simulink model "Microgrid"  (R2022b)
settings: Solver=ode45  StartTime=0.0  StopTime=0.5  RelTol=1e-3  EnableMultiTasking=on
model workspace (MAT data in the model file):
  AFPV = 1
  AFW = 1
  DG = 1
  pvc = 1
  wf1 = 1
undefined symbols (not defined in the file): BMSS1, D1, Delta, Ion, Lithium, R
libraries: spsDiodeLib x10, spsVoltageMeasurementLib x8, spsThreePhaseVIMeasurementLib x7, spsSeriesRLCBranchLib x7, fuzblock x6, spsMosfetLib x3, powerlib_extras x3, spsBreakerLib x2, spsThreePhaseParallelRLCLoadLib x2, spsThreePhaseBreakerLib x2, spsPWMGenerator2LevelLib x2, spsBatteryLib x1
(part 1 of 2)
settings Model: Creator=Indhu  LastModifiedBy=zs
settings SolverCC: AlgebraicLoopSolver=TrustRegion
settings DataIOCC: LimitDataPoints=on  SaveFormat=Array  ReturnWorkspaceOutputs=off
settings OptimizationCC: LifeSpan=inf
settings DebuggingCC: SolverPrmCheckMsg=warning  UnconnectedInputMsg=warning  UnconnectedOutputMsg=warning  UnconnectedLineMsg=warning  SFUnexpectedBacktrackingDiag=warning  SFNoUnconditionalDefaultTransitionDiag=warning  SFExecutionAtInitializationDiag=none  SFMachineParentedDataDiag=warning  ArithmeticOperatorsInVariantConditions=warning
settings HardwareCC: ProdBitPerPointer=32  ProdBitPerSizeT=32  ProdBitPerPtrDiffT=32  ProdLargestAtomicFloat=None  ProdIntDivRoundTo=Undefined  ProdEndianess=Unspecified  ProdWordSize=32  ProdHWDeviceType=32-bit Generic
settings ModelReferenceCC: EnableRefExpFcnMdlSchedulingChecks=on  PropagateSignalLabelsOutOfModel=off
settings SFSimCC: SimUseLocalCustomCode=off  CustomCodeUndefinedFunction=UseInterfaceOnly
settings RTWCC: RTWUseLocalCustomCode=off
settings CodeAppCC: StateflowObjectComments=on
settings GRTTargetCC: TargetLangStandard=C89/C90 (ANSI)
settings ConfigComp: CovMetricSettings=dw  CovSaveCumulativeToWorkspaceVar=on  CovSaveSingleToWorkspaceVar=on  CovExternalEMLEnable=off  CovSFcnEnable=off
settings SimscapeCC: SimscapeNormalizeSystem=off

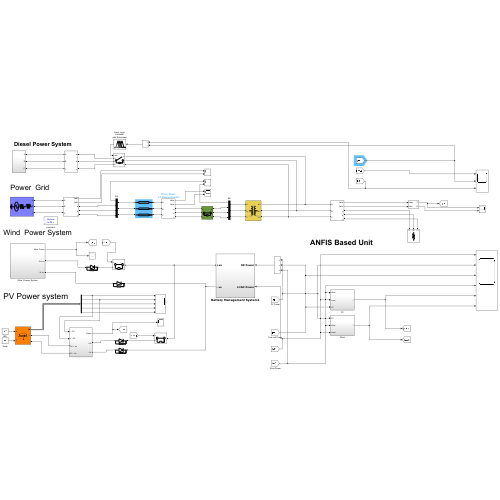
[thumbnail: Simulink's stored preview of the top-level diagram]
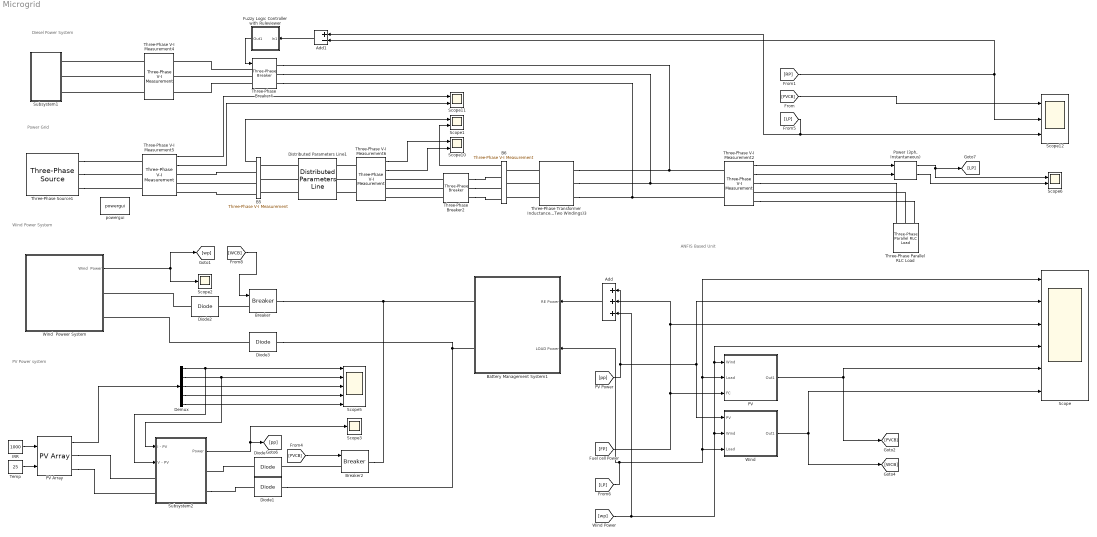
== system Microgrid ==
  note: ANFIS Based Unit
  note: Power Grid
  note: Wind Power System
  note: PV Power system
  note: Diesel Power System
  Add : Sum  Inputs=+++
  Add1 : Sum  Inputs=+-
  B5 : spsThreePhaseVIMeasurementLib/Three-Phase V-I Measurement  VoltageMeasurement=phase-to-ground  SetLabelV=off  LabelV=Vabc_B12  Vpu=off  VpuLL=off  CurrentMeasurement=no  SetLabelI=off  LabelI=A1  Ipu=off  Pbase=100e6  Vbase=25e3  OutputType=Magnitude  PhasorSimulation=off  PSBequivalent=0
  B6 : spsThreePhaseVIMeasurementLib/Three-Phase V-I Measurement  VoltageMeasurement=phase-to-phase  SetLabelV=off  LabelV=Vabc_B12  Vpu=off  VpuLL=off  CurrentMeasurement=no  SetLabelI=off  LabelI=A1  Ipu=off  Pbase=100e6  Vbase=440  OutputType=Magnitude  PhasorSimulation=off  PSBequivalent=0
  Battery Management System1 : Subsystem
  Breaker : spsBreakerLib/Breaker  InitialState=1  SwitchingTimes="[1/60  5/60]"  External=on  BreakerResistance=0.01  SnubberResistance=1e6  SnubberCapacitance=inf  Measurements=None  MoreParameters=on  NoBreakLoop=off
  Breaker2 : spsBreakerLib/Breaker  InitialState=1  SwitchingTimes="[1/60  5/60]"  External=on  BreakerResistance=0.01  SnubberResistance=1e6  SnubberCapacitance=inf  Measurements=None  MoreParameters=on  NoBreakLoop=off
  Demux : Demux  Outputs=5
  Diode{,1..3} (4 alike) : spsDiodeLib/Diode  Ron=0.001  Lon=0  Vf=0.8  IC=0  UseSnubber=off  Rs=500  Cs=250e-9  Measurements=off
  Distributed Parameters Line1 : spsDistributedParametersLineLib/Distributed Parameters Line  Phases=3  Length=100  Frequency=50  Resistance=[0.01273 0.3864]  Inductance="[0.9337e-3  4.1264e-3]"  Capacitance=[12.74e-9 7.751e-9]  x1=[-0.000566 2.77076590585873e-09 21709.9833530794 -60790.4116423668;-0.000565 2.76912057824268e-09 21729.080152483 -60783.5882501713;-0.000564 2.76747497732538e-09 21748.1748073123 -60776.7588588762;-0.000563 2.76582910326925e-09 21767.2673156828 -60769.9234691554;-0.000562 2.76418295623673e-09 21786.3576757102 -60763.0820816836;-0.000561 2.76253653639029e-09 21805.4458855103 -60756.234697136;-0.00056 2.76088984389243e-09 21824.5319431991 -60749.3813161885;-0.000559 2.75924287890566e-09 21843.615846893 -60742.5219395174;-0.000558 2.75759564159254e-09 21862.6975947085 -60735.6565677998;-0.000557 2.75594813211564e-09 21881.7771847622 -60728.7852017131;-0.000556 2.75430035063756e-09 21900.8546151711 -60721.9078419357;-0.000555 2.75265229732094e-09 21919.9298840522 -60715.0244891462;-0.000554 2.75100397232843e-09 21939.0029895231 -60708.1351440241;-0.000553 2.74935537582271e-09 21958.0739297011 -60701.2398072492;-0.000552 2.74770650796649e-09 21977.1427027041 -60694.3384795021;-0.000551 2.74605736892252e-09 21996.2093066501 -60687.431161464;-0.00055 2.74440795885354e-09 22015.2737396573 -60680.5178538165;-0.000549 2.74275827792236e-09 22034.3359998441 -60673.598557242;-0.000548 2.74110832629179e-09 22053.3960853291 -60666.6732724235;-0.000547 2.73945810412468e-09 22072.4539942312 -60659.7420000443;-0.000546 2.73780761158389e-09 22091.5097246694 -60652.8047407886;-0.000545 2.73615684883232e-09 22110.5632747629 -60645.8614953411;-0.000544 2.7345058160329e-09 22129.6146426314 -60638.912264387;-0.000543 2.73285451334857e-09 22148.6638263945 -60631.9570486122;-0.000542 2.73120294094231e-09 22167.7108241721 -60624.9958487031;-0.000541 2.72955109897714e-09 22186.7556340844 -60618.0286653468;-0.00054 2.72789898761607e-09 22205.7982542516 -60611.055499231;-0.000539 2.72624660702216e-09 22224.8386827945 -60604.0763510438;-0.000538 2.7245939573585e-09 22243.8769178337 -60597.0912214741;-0.000537 2.72294103878819e-09 22262.9129574902 -60590.1001112112;-0.000536 2.72128785147438e-09 22281.9467998854 -60583.1030209452;-0.000535 2.71963439558023e-09 22300.9784431405 -60576.0999513666;-0.000534 2.71798067126893e-09 22320.0078853774 -60569.0909031667;-0.000533 2.71632667870368e-09 22339.0351247177 -60562.0758770372;-0.000532 2.71467241804774e-09 22358.0601592837 -60555.0548736704;-0.000531 2.71301788946438e-09 22377.0829871976 -60548.0278937593;-0.00053 2.71136309311688e-09 22396.103606582 -60540.9949379974;-0.000529 2.70970802916857e-09 22415.1220155596 -60533.9560070788;-0.000528 2.70805269778281e-09 22434.1382122533 -60526.9111016984;-0.000527 2.70639709912295e-09 22453.1521947863 -60519.8602225512;-0.000526 2.70474123335242e-09 22472.1639612821 -60512.8033703334;-0.000525 2.70308510063462e-09 22491.1735098642 -60505.7405457413;-0.000524 2.70142870113302e-09 22510.1808386564 -60498.671749472;-0.000523 2.6997720350111e-09 22529.1859457829 -60491.5969822232;-0.000522 2.69811510243236e-09 22548.1888293679 -60484.5162446931;-0.000521 2.69645790356033e-09 22567.1894875358 -60477.4295375806;-0.00052 2.69480043855858e-09 22586.1879184115 -60470.3368615851;-0.000519 2.69314270759069e-09 22605.1841201197 -60463.2382174066;-0.000518 2.69148471082027e-09 22624.1780907858 -60456.1336057458;-0.000517 2.68982644841096e-09 22643.1698285349 -60449.0230273037;-0.000516 2.68816792052642e-09 22662.1593314929 -60441.9064827823;-0.000515 2.68650912733035e-09 22681.1465977853 -60434.7839728839;-0.000514 2.68485006898645e-09 22700.1316255383 -60427.6554983114;-0.000513 2.68319074565847e-09 22719.1144128782 -60420.5210597684;-0.000512 2.68153115751019e-09 22738.0949579314 -60413.3806579591;-0.000511 2.67987130470539e-09 22757.0732588245 -60406.2342935881;-0.00051 2.67821118740789e-09 22776.0493136846 -60399.0819673609;-0.000509 2.67655080578155e-09 22795.0231206387 -60391.9236799832;-0.000508 2.67489015999024e-09 22813.9946778142 -60384.7594321616;-0.000507 2.67322925019785e-09 22832.9639833388 -60377.5892246032;-0.000506 2.67156807656831e-09 22851.9310353401 ...(+33013 chars)]  x2=[-0.000566 1.4309886308804e-08 21803.469224195 -61159.1015753649;-0.000565 1.43032919359107e-08 21822.6818463418 -61152.2487955231;-0.000564 1.42966961513391e-08 21841.8923146763 -61145.3899801964;-0.000563 1.42900989557401e-08 21861.1006273024 -61138.5251300616;-0.000562 1.4283500349765e-08 21880.3067823244 -61131.6542457963;-0.000561 1.42769003340648e-08 21899.5107778466 -61124.7773280786;-0.00056 1.42702989092911e-08 21918.7126119739 -61117.8943775873;-0.000559 1.42636960760953e-08 21937.9122828109 -61111.0053950016;-0.000558 1.42570918351292e-08 21957.1097884627 -61104.1103810014;-0.000557 1.42504861870445e-08 21976.3051270348 -61097.2093362674;-0.000556 1.42438791324932e-08 21995.4982966324 -61090.3022614805;-0.000555 1.42372706721274e-08 22014.6892953614 -61083.3891573226;-0.000554 1.42306608065993e-08 22033.8781213277 -61076.4700244758;-0.000553 1.42240495365613e-08 22053.0647726374 -61069.5448636231;-0.000552 1.42174368626659e-08 22072.2492473968 -61062.6136754479;-0.000551 1.42108227855658e-08 22091.4315437126 -61055.6764606344;-0.00055 1.42042073059136e-08 22110.6116596915 -61048.7332198672;-0.000549 1.41975904243625e-08 22129.7895934406 -61041.7839538316;-0.000548 1.41909721415653e-08 22148.9653430669 -61034.8286632135;-0.000547 1.41843524581753e-08 22168.138906678 -61027.8673486993;-0.000546 1.41777313748458e-08 22187.3102823816 -61020.900010976;-0.000545 1.41711088922304e-08 22206.4794682854 -61013.9266507313;-0.000544 1.41644850109825e-08 22225.6464624975 -61006.9472686536;-0.000543 1.41578597317561e-08 22244.8112631263 -60999.9618654315;-0.000542 1.41512330552049e-08 22263.9738682802 -60992.9704417545;-0.000541 1.4144604981983e-08 22283.134276068 -60985.9729983127;-0.00054 1.41379755127446e-08 22302.2924845986 -60978.9695357967;-0.000539 1.41313446481439e-08 22321.4484919811 -60971.9600548976;-0.000538 1.41247123888354e-08 22340.6022963251 -60964.9445563074;-0.000537 1.41180787354737e-08 22359.75389574 -60957.9230407183;-0.000536 1.41114436887135e-08 22378.9032883356 -60950.8955088235;-0.000535 1.41048072492097e-08 22398.0504722221 -60943.8619613164;-0.000534 1.40981694176171e-08 22417.1954455096 -60936.8223988913;-0.000533 1.40915301945911e-08 22436.3382063086 -60929.7768222429;-0.000532 1.40848895807867e-08 22455.4787527297 -60922.7252320667;-0.000531 1.40782475768595e-08 22474.617082884 -60915.6676290585;-0.00053 1.4071604183465e-08 22493.7531948826 -60908.604013915;-0.000529 1.40649594012588e-08 22512.8870868366 -60901.5343873333;-0.000528 1.40583132308967e-08 22532.0187568578 -60894.4587500111;-0.000527 1.40516656730348e-08 22551.1482030579 -60887.3771026467;-0.000526 1.40450167283291e-08 22570.2754235489 -60880.2894459392;-0.000525 1.40383663974358e-08 22589.4004164431 -60873.1957805879;-0.000524 1.40317146810112e-08 22608.5231798528 -60866.0961072932;-0.000523 1.4025061579712e-08 22627.6437118907 -60858.9904267555;-0.000522 1.40184070941947e-08 22646.7620106697 -60851.8787396764;-0.000521 1.4011751225116e-08 22665.8780743029 -60844.7610467575;-0.00052 1.4005093973133e-08 22684.9919009036 -60837.6373487015;-0.000519 1.39984353389026e-08 22704.1034885854 -60830.5076462114;-0.000518 1.3991775323082e-08 22723.212835462 -60823.3719399909;-0.000517 1.39851139263285e-08 22742.3199396474 -60816.2302307443;-0.000516 1.39784511492997e-08 22761.4247992558 -60809.0825191764;-0.000515 1.3971786992653e-08 22780.5274124017 -60801.9288059926;-0.000514 1.39651214570463e-08 22799.6277771996 -60794.7690918991;-0.000513 1.39584545431373e-08 22818.7258917645 -60787.6033776024;-0.000512 1.3951786251584e-08 22837.8217542114 -60780.4316638097;-0.000511 1.39451165830447e-08 22856.9153626557 -60773.253951229;-0.00051 1.39384455381776e-08 22876.0067152129 -60766.0702405685;-0.000509 1.3931773117641e-08 22895.0958099987 -60758.8805325374;-0.000508 1.39250993220935e-08 22914.1826451292 -60751.6848278452;-0.000507 1.39184241521939e-08 22933.2672187205 -60744.483127202;-0.000506 1.39117476086008e-08 22952.3495288891 -60737.2754313188 ...(+32992 chars)]  x3=[-0.000566 1.37069561345331e-10 55.3596099410286 -231.821785243805;-0.000565 1.37082432995365e-10 55.4324361696897 -231.804382069755;-0.000564 1.37095291115906e-10 55.5052569273886 -231.786956017529;-0.000563 1.37108135705683e-10 55.5780722069384 -231.769507088848;-0.000562 1.3712096676343e-10 55.6508820011523 -231.752035285434;-0.000561 1.37133784287881e-10 55.7236863028444 -231.734540609011;-0.00056 1.37146588277769e-10 55.7964851048291 -231.717023061306;-0.000559 1.37159378731832e-10 55.8692783999215 -231.699482644048;-0.000558 1.37172155648806e-10 55.9420661809372 -231.681919358967;-0.000557 1.37184919027432e-10 56.0148484406923 -231.664333207798;-0.000556 1.37197668866449e-10 56.0876251720036 -231.646724192275;-0.000555 1.37210405164599e-10 56.1603963676881 -231.629092314138;-0.000554 1.37223127920625e-10 56.2331620205637 -231.611437575125;-0.000553 1.37235837133271e-10 56.3059221234488 -231.59375997698;-0.000552 1.37248532801283e-10 56.3786766691621 -231.576059521448;-0.000551 1.37261214923408e-10 56.4514256505231 -231.558336210274;-0.00055 1.37273883498394e-10 56.5241690603518 -231.54059004521;-0.000549 1.37286538524991e-10 56.5969068914686 -231.522821028005;-0.000548 1.3729918000195e-10 56.6696391366947 -231.505029160413;-0.000547 1.37311807928023e-10 56.7423657888516 -231.487214444191;-0.000546 1.37324422301964e-10 56.8150868407616 -231.469376881098;-0.000545 1.37337023122528e-10 56.8878022852472 -231.451516472892;-0.000544 1.37349610388471e-10 56.9605121151319 -231.433633221338;-0.000543 1.37362184098551e-10 57.0332163232394 -231.4157271282;-0.000542 1.37374744251527e-10 57.1059149023942 -231.397798195245;-0.000541 1.37387290846159e-10 57.1786078454211 -231.379846424243;-0.00054 1.37399823881209e-10 57.2512951451456 -231.361871816966;-0.000539 1.37412343355441e-10 57.3239767943938 -231.343874375187;-0.000538 1.37424849267617e-10 57.3966527859924 -231.325854100684;-0.000537 1.37437341616505e-10 57.4693231127684 -231.307810995234;-0.000536 1.37449820400871e-10 57.5419877675496 -231.289745060618;-0.000535 1.37462285619484e-10 57.6146467431644 -231.27165629862;-0.000534 1.37474737271113e-10 57.6873000324414 -231.253544711024;-0.000533 1.37487175354529e-10 57.7599476282102 -231.235410299618;-0.000532 1.37499599868505e-10 57.8325895233007 -231.217253066193;-0.000531 1.37512010811815e-10 57.9052257105435 -231.199073012539;-0.00053 1.37524408183233e-10 57.9778561827696 -231.180870140452;-0.000529 1.37536791981537e-10 58.0504809328107 -231.162644451727;-0.000528 1.37549162205503e-10 58.123099953499 -231.144395948165;-0.000527 1.37561518853911e-10 58.1957132376674 -231.126124631564;-0.000526 1.37573861925542e-10 58.2683207781491 -231.10783050373;-0.000525 1.37586191419176e-10 58.3409225677781 -231.089513566468;-0.000524 1.37598507333598e-10 58.4135185993889 -231.071173821585;-0.000523 1.37610809667592e-10 58.4861088658166 -231.052811270891;-0.000522 1.37623098419944e-10 58.5586933598967 -231.034425916199;-0.000521 1.3763537358944e-10 58.6312720744655 -231.016017759323;-0.00052 1.37647635174869e-10 58.7038450023597 -230.997586802081;-0.000519 1.37659883175022e-10 58.7764121364167 -230.979133046291;-0.000518 1.37672117588688e-10 58.8489734694744 -230.960656493774;-0.000517 1.37684338414662e-10 58.9215289943713 -230.942157146354;-0.000516 1.37696545651736e-10 58.9940787039464 -230.923635005857;-0.000515 1.37708739298705e-10 59.0666225910393 -230.905090074112;-0.000514 1.37720919354367e-10 59.1391606484903 -230.886522352947;-0.000513 1.3773308581752e-10 59.2116928691402 -230.867931844196;-0.000512 1.37745238686961e-10 59.2842192458303 -230.849318549694;-0.000511 1.37757377961493e-10 59.3567397714025 -230.830682471277;-0.00051 1.37769503639917e-10 59.4292544386993 -230.812023610786;-0.000509 1.37781615721035e-10 59.5017632405639 -230.793341970061;-0.000508 1.37793714203654e-10 59.5742661698399 -230.774637550946;-0.000507 1.37805799086578e-10 59.6467632193716 -230.755910355288;-0.000506 1.37817870368614e-10 59.7192543820037 ...(+33006 chars)]  x4=[-0.000566 -1.1176625836894e-10 80.4359037202969 -225.752108293466;-0.000565 -1.11789344885578e-10 80.5068218662724 -225.72682746904;-0.000564 -1.11812420369049e-10 80.5777320665431 -225.70152436627;-0.000563 -1.11835484817077e-10 80.6486343141105 -225.676198987652;-0.000562 -1.11858538227385e-10 80.7195286019768 -225.650851335687;-0.000561 -1.11881580597698e-10 80.790414923145 -225.625481412875;-0.00056 -1.11904611925742e-10 80.861293270619 -225.600089221721;-0.000559 -1.11927632209243e-10 80.9321636374032 -225.574674764731;-0.000558 -1.1195064144593e-10 81.0030260165031 -225.549238044413;-0.000557 -1.11973639633531e-10 81.0738804009249 -225.523779063278;-0.000556 -1.11996626769778e-10 81.1447267836754 -225.498297823838;-0.000555 -1.120196028524e-10 81.2155651577625 -225.472794328608;-0.000554 -1.12042567879131e-10 81.2863955161947 -225.447268580106;-0.000553 -1.12065521847704e-10 81.3572178519813 -225.42172058085;-0.000552 -1.12088464755853e-10 81.4280321581323 -225.396150333363;-0.000551 -1.12111396601314e-10 81.4988384276588 -225.370557840167;-0.00055 -1.12134317381824e-10 81.5696366535725 -225.344943103789;-0.000549 -1.1215722709512e-10 81.6404268288857 -225.319306126757;-0.000548 -1.12180125738942e-10 81.7112089466118 -225.293646911601;-0.000547 -1.1220301331103e-10 81.781982999765 -225.267965460853;-0.000546 -1.12225889809124e-10 81.85274898136 -225.242261777048;-0.000545 -1.12248755230966e-10 81.9235068844125 -225.216535862724;-0.000544 -1.12271609574301e-10 81.9942567019392 -225.190787720418;-0.000543 -1.12294452836872e-10 82.064998426957 -225.165017352673;-0.000542 -1.12317285016425e-10 82.1357320524843 -225.139224762031;-0.000541 -1.12340106110707e-10 82.2064575715398 -225.113409951039;-0.00054 -1.12362916117464e-10 82.2771749771432 -225.087572922244;-0.000539 -1.12385715034446e-10 82.347884262315 -225.061713678196;-0.000538 -1.12408502859403e-10 82.4185854200764 -225.035832221448;-0.000537 -1.12431279590085e-10 82.4892784434496 -225.009928554553;-0.000536 -1.12454045224245e-10 82.5599633254574 -224.984002680069;-0.000535 -1.12476799759635e-10 82.6306400591235 -224.958054600554;-0.000534 -1.12499543194011e-10 82.7013086374724 -224.932084318569;-0.000533 -1.12522275525127e-10 82.7719690535293 -224.906091836677;-0.000532 -1.12544996750739e-10 82.8426213003204 -224.880077157444;-0.000531 -1.12567706868605e-10 82.9132653708726 -224.854040283437;-0.00053 -1.12590405876485e-10 82.9839012582135 -224.827981217226;-0.000529 -1.12613093772136e-10 83.0545289553718 -224.801899961383;-0.000528 -1.12635770553321e-10 83.1251484553766 -224.775796518481;-0.000527 -1.12658436217801e-10 83.1957597512583 -224.749670891099;-0.000526 -1.12681090763339e-10 83.2663628360476 -224.723523081812;-0.000525 -1.127037341877e-10 83.3369577027764 -224.697353093204;-0.000524 -1.12726366488647e-10 83.4075443444772 -224.671160927856;-0.000523 -1.12748987663949e-10 83.4781227541834 -224.644946588353;-0.000522 -1.12771597711371e-10 83.5486929249292 -224.618710077282;-0.000521 -1.12794196628683e-10 83.6192548497496 -224.592451397234;-0.00052 -1.12816784413654e-10 83.6898085216804 -224.5661705508;-0.000519 -1.12839361064055e-10 83.7603539337583 -224.539867540573;-0.000518 -1.12861926577657e-10 83.8308910790206 -224.513542369149;-0.000517 -1.12884480952234e-10 83.9014199505057 -224.487195039128;-0.000516 -1.12907024185559e-10 83.9719405412526 -224.460825553108;-0.000515 -1.12929556275407e-10 84.0424528443012 -224.434433913693;-0.000514 -1.12952077219556e-10 84.1129568526923 -224.408020123488;-0.000513 -1.12974587015781e-10 84.1834525594674 -224.381584185098;-0.000512 -1.12997085661861e-10 84.2539399576688 -224.355126101135;-0.000511 -1.13019573155576e-10 84.3244190403397 -224.328645874208;-0.00051 -1.13042049494707e-10 84.3948898005241 -224.302143506931;-0.000509 -1.13064514677034e-10 84.4653522312668 -224.27561900192;-0.000508 -1.13086968700342e-10 84.5358063256135 -224.249072361794;-0.000507 -1.13109411562413e-10 84.6062520766105 -224.222503589171 ...(+33567 chars)]  x5=0.000565541566995743  V1=[0 0 0 2.339e-09 6.456e+04 6.456e+04;0 0 0 314.2 314.2 314.2;1.571 1.571 1.571 -0.9334 0.4129 -1.158]  V2=[0 0 0 9.955e-09 6.494e+04 6.494e+04;0 0 0 314.2 314.2 314.2;1.571 1.571 1.571 -1.047 0.4126 -1.158]  I1=[0 0 0 5.638e-11 239 239;0 0 0 314.2 314.2 314.2;1.571 1.571 1.571 -2.312 0.3045 -1.266]  I2=[0 0 0 5.238e-11 239.1 239.1;0 0 0 314.2 314.2 314.2;1.571 1.571 1.571 0.5382 0.4125 -1.158]  nHarmo=2  Measurements=None  Decoupling=off  VsMag0=0  VrMag0=0  VsAngle0=0  VrAngle0=0  IsMag0=0  IrMag0=0  IsAngle0=0  IrAngle0=0
      settings: LibrarySourceBlock=sps_lib/Power Grid Elements/Distributed Parameters Line
  Fuzzy Logic Controller with Ruleviewer : Subsystem  AncestorBlock=|  mask(Fuzzy Inference System){fismatrix=[DG], Ts=0.01}
      | fuzblock/Fuzzy Logic 
      | Controller 
      | with Ruleviewer
      mask prompts: fismatrix "fuzzy:dialogs:flcWithRuleViewerMaskPrompt_paramFIS"; Ts "fuzzy:dialogs:flcWithRuleViewerMaskPrompt_paramRate"
      mask help: fuzzy:dialogs:flcWithRuleViewerMask_description
      mask init:
      | fuzzy.internal.utility.errorIfType2FIS(fismatrix)
      settings: LibrarySourceBlock=|
      | fuzblock/Fuzzy Logic
      | Controller
      | with Ruleviewer
      mask Help: helpview(fullfile(docroot,'toolbox','fuzzy','fuzzy.map'), 'fuzviewerblock');
      mask DialogControl DescGroupVar Prompt: Fuzzy Inference System
      mask DialogControl fismatrix Prompt: FIS structure:
      mask DialogControl Ts Prompt: Refresh rate (s):
      mask Display: plot(0, -0.3, 6, -0.3, 0, 1.2, 6, 1.2, [0 6], [0 0], [1 2 3],[0 1 0],[2 3 4],[0 1 0],[3 4 5],[0 1 0])
  IRR : Constant  Value=1000
  PV : Subsystem
  PV Array : spsPVArrayLib/PV Array  Npar=10  Nser=5  PlotType=array @ 25 deg.C & specified irradiances  S_vec="[ 1000  500  100 ]"  Temp_C_vec="[ 45 25  ]"  ModuleName=User-defined  PlotWhenSelected=off  Pm=334.905  Ncell=80  Voc=49.9  Isc=9  Vm=41.5  Im=8.07  beta_Voc_pc=-0.36  alpha_Isc_pc=0.09  beta_Voc=-0.17964  alpha_Isc=0.0081  IL=9.0297  I0=3.1312e-10  nI=1.0111  Rsh=77.6407  Rs=0.25633  RobustModel=off  RobustCellTemperature=313.3991  BAL=off  Tc=1e-6  Tfilter=5e-5
  "Power (3ph, Instantaneous)" : spsPower3phInstantaneousLib/Power (3ph, Instantaneous)
  Scope : Scope  NumInputPorts=6
  Scope{1,6,10..11} (4 alike) : Scope  NumInputPorts=2
  Scope12 : Scope  NumInputPorts=3
  Scope2 : Scope
  Scope3 : Scope
  Scope5 : Scope  NumInputPorts=5
  Subsystem1 : Subsystem
  Subsystem2 : Subsystem
  "Temp " : Constant  Value=25
  Three-Phase Parallel RLC Load : spsThreePhaseParallelRLCLoadLib/Three-Phase Parallel RLC Load  LConnTagsString=A|B|C  Configuration=Delta  NominalVoltage=400  Vabc=[1e3 1e3 1e3]  Vabcp=[1e3 1e3 1e3]  NominalFrequency=50  UnbalancedPower=off  ActivePower=100e3  InductivePower=0  CapacitivePower=0  Pabc=[10e3 9e3 11e3]  QLabc=[100 90 110]  QCabc=[100 90 110]  Pabcp=[10e3 9e3 11e3]  QLabcp=[100 90 110]  QCabcp=[100 90 110]  Measurements=Branch voltages and currents  LoadType=constant PQ
  Three-Phase V-I Measurement2 : spsThreePhaseVIMeasurementLib/Three-Phase V-I Measurement  VoltageMeasurement=phase-to-phase  SetLabelV=off  LabelV=Vabc_b1  Vpu=off  VpuLL=off  CurrentMeasurement=yes  SetLabelI=off  LabelI=Iabc_b1  Ipu=off  Pbase=100e6  Vbase=500e3  OutputType=Complex  PhasorSimulation=off  PSBequivalent=0
  Three-Phase V-I Measurement4 : spsThreePhaseVIMeasurementLib/Three-Phase V-I Measurement  VoltageMeasurement=no  SetLabelV=off  LabelV=Vabc_b1  Vpu=off  VpuLL=off  CurrentMeasurement=no  SetLabelI=off  LabelI=Iabc_b1  Ipu=off  Pbase=100e6  Vbase=500e3  OutputType=Complex  PhasorSimulation=off  PSBequivalent=0
  Three-Phase V-I Measurement5 : spsThreePhaseVIMeasurementLib/Three-Phase V-I Measurement  VoltageMeasurement=phase-to-ground  SetLabelV=off  LabelV=Vabc  Vpu=off  VpuLL=off  CurrentMeasurement=yes  SetLabelI=off  LabelI=Iabc  Ipu=off  Pbase=100e6  Vbase=500e3  OutputType=Complex  PhasorSimulation=off  PSBequivalent=0
  Three-Phase V-I Measurement6 : spsThreePhaseVIMeasurementLib/Three-Phase V-I Measurement  VoltageMeasurement=phase-to-ground  SetLabelV=off  LabelV=Vabc  Vpu=off  VpuLL=off  CurrentMeasurement=yes  SetLabelI=off  LabelI=Iabc  Ipu=off  Pbase=100e6  Vbase=500e3  OutputType=Complex  PhasorSimulation=off  PSBequivalent=0
  Three-Phase Breaker2 : spsThreePhaseBreakerLib/Three-Phase Breaker  InitialState=closed  SwitchA=off  SwitchB=off  SwitchC=off  SwitchTimes="[1/50  20/50]"  External=off  BreakerResistance=0.001  SnubberResistance=1e6  SnubberCapacitance=inf  Measurements=None
  Three-Phase Breaker4 : spsThreePhaseBreakerLib/Three-Phase Breaker  InitialState=open  SwitchA=on  SwitchB=on  SwitchC=on  SwitchTimes=[0.02 1]  External=on  BreakerResistance=0.01  SnubberResistance=1e6  SnubberCapacitance=inf  Measurements=None
  Three-Phase Source1 : spsThreePhaseSourceLib/Three-Phase Source  InternalConnection=Yg  VoltagePhases=off  Voltage=63510.4  PhaseAngle=0  Voltage_phases=[25e3 25e3 25e3]/sqrt(3)  PhaseAngles_phases=[0 -120 +120]  Frequency=50  NonIdealSource=on  SpecifyImpedance=on  Resistance=0.8929  Inductance=16.58e-3  ShortCircuitLevel=100e6  BaseVoltage=63510.4  XRratio=7  BusType=swing  Pref=0  Qref=0  Prefabc=[10e3, 10e3, 10e3]  Qrefabc=[0, 0, 0]  Qmin=-inf  Qmax=inf
  Three-Phase Transformer Inductance Matrix Type (Two Windings)3 : spsThreePhaseTransformerInductanceMatrixTypeTwoWindingsLib/Three-Phase Transformer Inductance Matrix Type (Two Windings)  CoreType=Three-limb or five-limb core  Winding1Connection=Delta (D1)  Winding2Connection=Delta (D1)  AutoTransformer=off  Measurements=None  NominalPower=[100e3 50]  VLLnom=[63510.4 254.03]  WindingResistances=[0.01 0.01]  NoLoadIexcPos=2  NoLoadPlossPos=1000  ShortCircuitReactancePos=0.06  ShortCircuitReactancePosAuto=0.06  NoLoadIexcZero=100  NoLoadPlossZero=1500  ShortCircuitReactanceZero=0.03  ShortCircuitReactanceZeroAuto=0.03
      settings: LibrarySourceBlock=|
      | sps_lib/Power Grid Elements/Three-Phase Transformer
      | Inductance Matrix Type
      | (Two Windings)
  Wind : Subsystem
  Wind  Poweer System : Subsystem
  powergui : sps_lib/powergui  Priority=1  SimulationMode=Discrete  SampleTime=1e-6  frequency=60  Iterations=50  frequencyindice=0  Pbase=100e6  ErrMax=1e-4  UnitsV=kV  UnitsW=MW  buscounter=0  FunctionMessages=off  echomessages=off  EnableUseOfTLC=off  CurrentSourceSwitches=off  DisableSnubberDevices=off  DisableRonSwitches=off  DisableVfSwitches=off  DisplayEquations=off  AutomaticDiscreteSolvers=off  SolverType=Tustin  Interpol=off  ExternalGateDelay=off  methode=off  Ts=0  x0status=blocks  SPID=off  SwTol=0  HookPort=off  NonlinearTolerance=1e-4  nMaxIteration=100  ContinueOnMaxIteration=off  RestoreLinks=warning  ResistiveCurrentMeasurement=off  Frange=[0:2:500]  Ylog=off  Xlog=on  ShowGrid=off  save=off  variable=ZData  structure=ScopeData4  ZoomFFT=off  StartTime=0.1  cycles=3  DisplayStyle=1  fundamental=50  FreqAxis=off  MaxFrequency=1000  frequencyindicesteady=1  RmsSteady=1  display=off
  wires:
  Three-Phase V-I Measurement6/1 -> Scope10/1
  Three-Phase V-I Measurement6/2 -> Scope10/2
  Three-Phase V-I Measurement5/1 -> Scope11/1
  Three-Phase V-I Measurement5/2 -> Scope11/2
  Demux/5 -> Scope5/5
  Demux/4 -> Scope5/4
  Demux/1 -> Subsystem2/2(V - PV), Scope5/1
  Demux/3 -> Scope5/3
  Demux/2 -> Subsystem2/1(I - PV), Scope5/2
  PV Array/1 -> Demux/1
  "Temp "/1 -> PV Array/2
  IRR/1 -> PV Array/1
  Subsystem2/1(Power) -> Scope3/1, [pp]
  Wind  Poweer System/1(Wind  Power) -> Scope2/1, [wp]
  Three-Phase V-I Measurement2/1 -> "Power (3ph, Instantaneous)"/1
  Three-Phase V-I Measurement2/2 -> "Power (3ph, Instantaneous)"/2
  [PVCB] -> Breaker2/1
  [WCB] -> Breaker/1
  PV/1(Out1) -> [PVCB], Scope/5
  [LP] -> Battery Management System1/2(LOAD Power), Wind/3(Load), PV/2(Load), Scope/1
  [pp] -> Wind/1(PV), Scope/2, Add/1
  [wp] -> Scope/4, PV/1(Wind), Wind/2(Wind), Add/3
  Wind/1(Out1) -> [WCB], Scope/6
  [FP] -> Add/2, Scope/3, PV/3(FC)
  Add/1 -> Battery Management System1/1(RE Power)
  "Power (3ph, Instantaneous)"/2 -> Scope6/2
  "Power (3ph, Instantaneous)"/1 -> [LP], Scope6/1
  [PVCB] -> Scope12/1
  [RP] -> Scope12/2, Add1/2
  [LP] -> Add1/1, Scope12/3
  Add1/1 -> Fuzzy Logic Controller with Ruleviewer/1(In1)
  Fuzzy Logic Controller with Ruleviewer/1(Out1) -> Three-Phase Breaker4/1
  B6/1 -> Scope1/2
  B5/1 -> Scope1/1
  connections:
  Three-Phase Breaker2/LConn3 -- B6/RConn3
  Three-Phase V-I Measurement6/LConn1 -- Distributed Parameters Line1/RConn1
  Three-Phase Transformer Inductance Matrix Type (Two Windings)3/LConn1 -- B6/LConn1
  B5/RConn1 -- Three-Phase V-I Measurement5/RConn1
  Three-Phase Source1/RConn3 -- Three-Phase V-I Measurement5/LConn3
  Three-Phase Breaker2/RConn1 -- Three-Phase V-I Measurement6/RConn1
  Three-Phase Source1/RConn1 -- Three-Phase V-I Measurement5/LConn1
  Three-Phase V-I Measurement6/LConn2 -- Distributed Parameters Line1/RConn2
  Three-Phase Transformer Inductance Matrix Type (Two Windings)3/LConn3 -- B6/LConn3
  Three-Phase Breaker2/LConn1 -- B6/RConn1
  Three-Phase Breaker2/LConn2 -- B6/RConn2
  Three-Phase Breaker2/RConn2 -- Three-Phase V-I Measurement6/RConn2
  Three-Phase V-I Measurement6/LConn3 -- Distributed Parameters Line1/RConn3
  Three-Phase Transformer Inductance Matrix Type (Two Windings)3/LConn2 -- B6/LConn2
  Distributed Parameters Line1/LConn1 -- B5/LConn1
  B5/RConn2 -- Three-Phase V-I Measurement5/RConn2
  Distributed Parameters Line1/LConn2 -- B5/LConn2
  Distributed Parameters Line1/LConn3 -- B5/LConn3
  B5/RConn3 -- Three-Phase V-I Measurement5/RConn3
  Three-Phase Breaker2/RConn3 -- Three-Phase V-I Measurement6/RConn3
  Three-Phase Source1/RConn2 -- Three-Phase V-I Measurement5/LConn2
  Three-Phase Breaker4/RConn1 -- Three-Phase V-I Measurement2/LConn1 -- Three-Phase Transformer Inductance Matrix Type (Two Windings)3/RConn1
  Three-Phase Breaker4/RConn3 -- Three-Phase V-I Measurement2/LConn3 -- Three-Phase Transformer Inductance Matrix Type (Two Windings)3/RConn3
  Three-Phase Breaker4/RConn2 -- Three-Phase V-I Measurement2/LConn2 -- Three-Phase Transformer Inductance Matrix Type (Two Windings)3/RConn2
  Diode/LConn1 -- Subsystem2/RConn1
  Subsystem2/RConn2 -- Diode1/LConn1
  PV Array/RConn1 -- Subsystem2/LConn1
  PV Array/RConn2 -- Subsystem2/LConn2
  Battery Management System1/RConn1 -- Breaker2/RConn1 -- Breaker/RConn1
  Diode1/RConn1 -- Diode3/RConn1 -- Battery Management System1/RConn2
  Diode2/LConn1 -- Wind  Poweer System/RConn1
  Diode3/LConn1 -- Wind  Poweer System/RConn2
  Breaker/LConn1 -- Diode2/RConn1
  Breaker2/LConn1 -- Diode/RConn1
  Three-Phase V-I Measurement2/RConn1 -- Three-Phase Parallel RLC Load/LConn1
  Three-Phase Parallel RLC Load/LConn2 -- Three-Phase V-I Measurement2/RConn2
  Three-Phase V-I Measurement2/RConn3 -- Three-Phase Parallel RLC Load/LConn3
  Three-Phase V-I Measurement4/LConn1 -- Subsystem1/RConn1
  Three-Phase Breaker4/LConn2 -- Three-Phase V-I Measurement4/RConn2
  Three-Phase Breaker4/LConn1 -- Three-Phase V-I Measurement4/RConn1
  Three-Phase V-I Measurement4/LConn3 -- Subsystem1/RConn3
  Three-Phase Breaker4/LConn3 -- Three-Phase V-I Measurement4/RConn3
  Three-Phase V-I Measurement4/LConn2 -- Subsystem1/RConn2
